simulink model "pend_state_estimator"  (Simulink 7.4)
settings: Solver=ode4  StartTime=0.0  StopTime=50  FixedStep=0.01  RelTol=1e-3
values from neighbouring files (symbols this model uses):
  a = J1 + m2*l1^2    (= 0.0264875)    [pend_lqr_init.m]
  As = [0   1.0000          0         0 ... (first row only)    [pend_lqr_init.m]
  b = m2*l1*l2    (= 0.001665)    [pend_lqr_init.m]
  Bs = [0;   2.2203;   0;  0.6718]    [pend_lqr_init.m]
  c = m2*l2^2    (= 0.0016428)    [pend_lqr_init.m]
  c2 = 2.8*10^-3    (= 0.0028)    [pend_lqr_init.m]
  d = Kt*Ke/Ra + c1    (= 0.00529230769231)    [pend_lqr_init.m]
  f = J2 + m2*l2^2    (= 0.0055028)    [pend_lqr_init.m]
  h = m2*g*l2    (= 0.10878)    [pend_lqr_init.m]
  K = lqr(As,Bs,Q,R)    [pend_lqr_init.m]    (also in pend_swingup_lqr_init.m)
undefined symbols (not defined in the file or in its folder): Cm, Cs, Lo
settings Model: Creator=User  LastModifiedBy=Administrator
settings OptimizationCC: InitFltsAndDblsToZero=on
settings DebuggingCC: SaveWithParameterizedLinksMsg=none  SignalResolutionControl=TryResolveAllWithWarning  MultiTaskDSMMsg=warning  MultiTaskCondExecSysMsg=none
settings RTWCC: IncludeERTFirstTime=on
settings GRTTargetCC: TargetFcnLib=ansi_tfl_tmw.mat

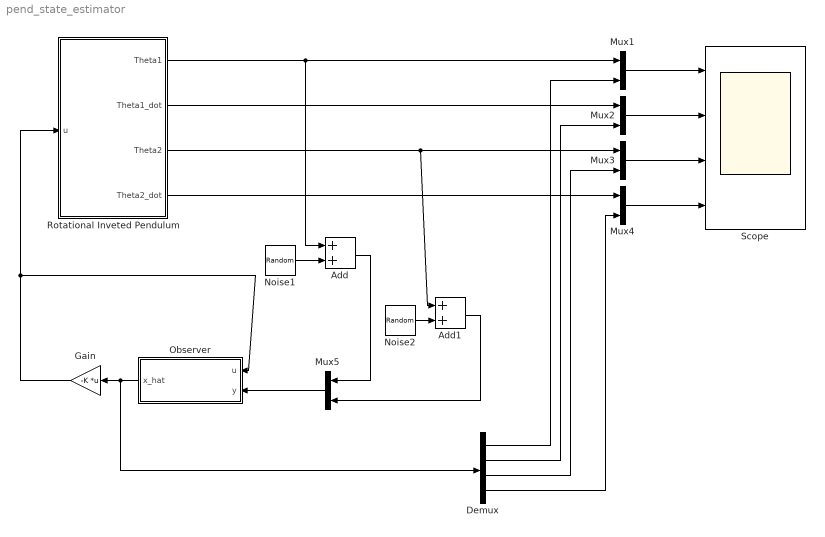
== system pend_state_estimator ==
  Add : Sum  OutDataType=sfix(16)  OutScaling=2^-10
  Add1 : Sum  OutDataType=sfix(16)  OutScaling=2^-10
  Demux : Demux
  Gain : Gain  Gain=-K  Multiplication=Matrix(K*u)  ParameterDataType=sfix(16)  ParameterScaling=2^0  OutDataType=sfix(16)  OutScaling=2^0
  Mux{1..5} (5 alike) : Mux  Inputs=2
  Noise1 : RandomNumber  Variance=0.001  SampleTime=0
  Noise2 : RandomNumber  Variance=0.001  SampleTime=0
  Observer : Subsystem
  Rotational Inveted Pendulum : Subsystem
  Scope : Scope  NumInputPorts=4
      settings: YMin=-5~-5~-5~-5  YMax=5~5~5~5
  wires:
  Gain/1 -> Observer/1(u), Rotational Inveted Pendulum/1(u)
  Noise1/1 -> Add/2
  Noise2/1 -> Add1/2
  Mux1/1 -> Scope/1
  Mux2/1 -> Scope/2
  Mux3/1 -> Scope/3
  Mux4/1 -> Scope/4
  Rotational Inveted Pendulum/1(Theta1) -> Mux1/1, Add/1
  Rotational Inveted Pendulum/2(Theta1_dot) -> Mux2/1
  Rotational Inveted Pendulum/3(Theta2) -> Mux3/1, Add1/1
  Rotational Inveted Pendulum/4(Theta2_dot) -> Mux4/1
  Add/1 -> Mux5/1
  Add1/1 -> Mux5/2
  Observer/1(x_hat) -> Gain/1, Demux/1
  Mux5/1 -> Observer/2(y)
  Demux/1 -> Mux1/2
  Demux/2 -> Mux2/2
  Demux/3 -> Mux3/2
  Demux/4 -> Mux4/2

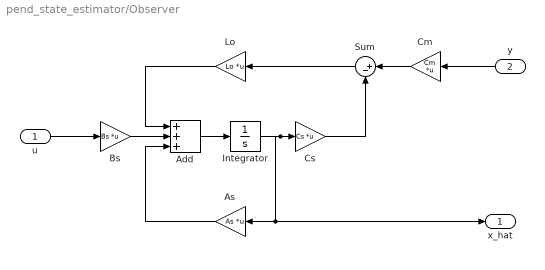
== system pend_state_estimator/Observer ==
  u : Inport  OutDataType=sfix(16)  OutScaling=2^0
  y : Inport  Port=2  OutDataType=sfix(16)  OutScaling=2^0
  Add : Sum  Inputs=+++  OutDataType=sfix(16)  OutScaling=2^-10
  As : Gain  Gain=As  Multiplication=Matrix(K*u)  ParameterDataType=sfix(16)  ParameterScaling=2^0  OutDataType=sfix(16)  OutScaling=2^0
  Bs : Gain  Gain=Bs  Multiplication=Matrix(K*u)  ParameterDataType=sfix(16)  ParameterScaling=2^0  OutDataType=sfix(16)  OutScaling=2^0
  Cm : Gain  Gain=Cm  Multiplication=Matrix(K*u)  ParameterDataType=sfix(16)  ParameterScaling=2^0  OutDataType=sfix(16)  OutScaling=2^0
  Cs : Gain  Gain=Cs  Multiplication=Matrix(K*u)  ParameterDataType=sfix(16)  ParameterScaling=2^0  OutDataType=sfix(16)  OutScaling=2^0
  Integrator : Integrator
  Lo : Gain  Gain=Lo  Multiplication=Matrix(K*u)  ParameterDataType=sfix(16)  ParameterScaling=2^0  OutDataType=sfix(16)  OutScaling=2^0
  Sum : Sum  Inputs=|+-  OutDataType=sfix(16)  OutScaling=2^0
  x_hat : Outport  OutDataType=sfix(16)  OutScaling=2^0
  wires:
  u/1 -> Bs/1
  Bs/1 -> Add/2
  Add/1 -> Integrator/1
  Lo/1 -> Add/1
  Integrator/1 -> Cs/1, As/1, x_hat/1
  Sum/1 -> Lo/1
  Cs/1 -> Sum/2
  Cm/1 -> Sum/1
  y/1 -> Cm/1
  As/1 -> Add/3

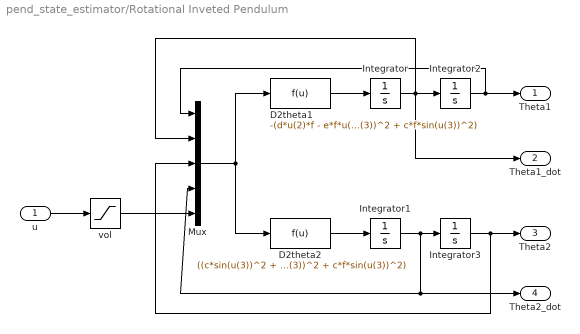
== system pend_state_estimator/Rotational Inveted Pendulum ==
  u : Inport  OutDataType=fixdt(1, 16)  OutScaling=2^0
  D2theta1 : Fcn  Expr=-(d*u(2)*f - e*f*u(5) + b*c2*u(4)*cos(u(3)) + b*u(4)^2*f*sin(u(3)) - b*h*cos(u(3))*sin(u(3)) - b*c*u(2)^2*cos(u(3))^2*sin(u(3)) + 2*c*u(2)*u(4)*f*cos(u(3))*sin(u(3)))/(a*f - b^2*cos(u(3))^2 + c*f*sin(u(3))^2)
  D2theta2 : Fcn  Expr=((c*sin(u(3))^2 + a)*((c*sin(2*u(3))*u(2)^2)/2 - c2*u(4) + h*sin(u(3))))/(a*f - b^2*cos(u(3))^2 + c*f*sin(u(3))^2) - (b*cos(u(3))*(b*sin(u(3))*u(4)^2 + c*u(2)*sin(2*u(3))*u(4) + d*u(2) - e*u(5)))/(a*f - b^2*cos(u(3))^2 + c*f*sin(u(3))^2)
  Integrator : Integrator
  Integrator1 : Integrator
  Integrator2 : Integrator
  Integrator3 : Integrator  InitialCondition=(pi/180)*10
  Mux : Mux  Inputs=5
  vol : Saturate  UpperLimit=25  LowerLimit=-25  OutDataType=fixdt(1, 16)  OutScaling=2^0
  Theta1 : Outport  OutDataType=fixdt(1, 16)  OutScaling=2^0
  Theta1_dot : Outport  Port=2  OutDataType=fixdt(1, 16)  OutScaling=2^0
  Theta2 : Outport  Port=3  OutDataType=fixdt(1, 16)  OutScaling=2^0
  Theta2_dot : Outport  Port=4  OutDataType=fixdt(1, 16)  OutScaling=2^0
  wires:
  u/1 -> vol/1
  Integrator2/1 -> Theta1/1, Mux/1
  Mux/1 -> D2theta1/1, D2theta2/1
  vol/1 -> Mux/5
  D2theta1/1 -> Integrator/1
  Integrator/1 -> Integrator2/1, Theta1_dot/1, Mux/2
  D2theta2/1 -> Integrator1/1
  Integrator1/1 -> Integrator3/1, Theta2_dot/1, Mux/4
  Integrator3/1 -> Theta2/1, Mux/3
